simulink model "twotanks_FMINUNC"  (R2017a)
settings: Solver=FixedStepAuto  StartTime=0.0  StopTime=150  FixedStep=0.1  RelTol=1e-3
values from neighbouring files (symbols this model uses):
  q = [1,1]    [MPC_RODAR_PRIMEIRO.m]
  r = [0.0001/(u1^2),0.0001/(u2^2)]    [MPC_RODAR_PRIMEIRO.m]
  Vd = 0.00001*eye(nx)    [MPC_RODAR_PRIMEIRO.m]
  Vn = 0.00001*eye(ny)    [MPC_RODAR_PRIMEIRO.m]
undefined symbols (not defined in the file or in its folder): sysi1, sysi2
libraries: simulink x2
settings Model: Creator=shpac  LastModifiedBy=aguia

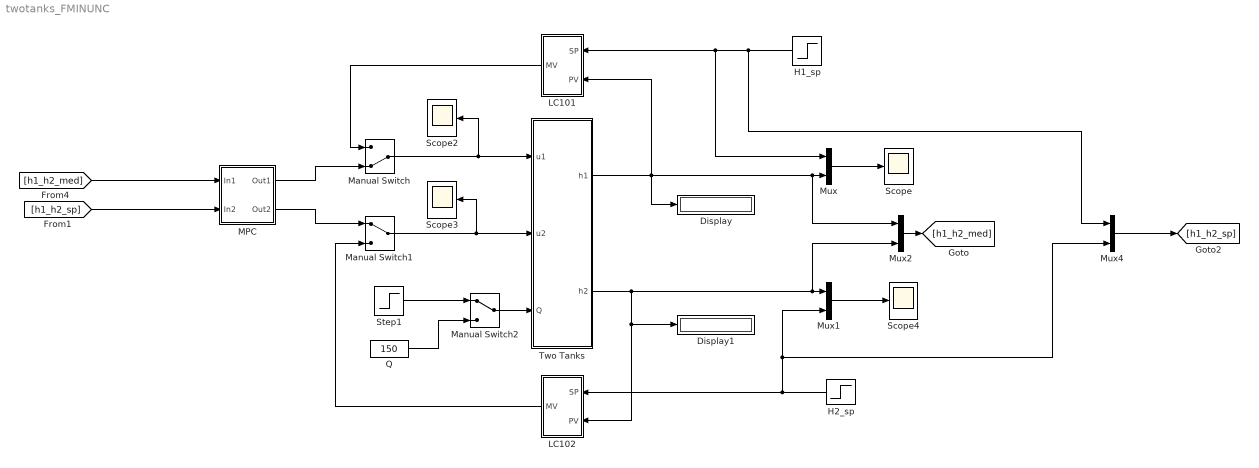
== system twotanks_FMINUNC ==
  Display : Display
  Display1 : Display
  H1_sp : Step  Time=120  Before=0.65  After=0.35  SampleTime=0
  H2_sp : Step  Time=20  Before=0.28  After=0.678  SampleTime=0
  LC101 : Subsystem
  LC102 : Subsystem
  MPC : Subsystem
  Manual Switch : ManualSwitch  CurrentSetting=0
  Manual Switch1 : ManualSwitch
  Manual Switch2 : ManualSwitch
  Mux{,1..2,4} (4 alike) : Mux  Inputs=2
  Q : Constant  Value=150
  Scope{,2..4} (4 alike) : Scope
  Step1 : Step  Time=70  Before=150  After=30  SampleTime=0
  Two Tanks : Subsystem
  wires:
  MPC/1(Out1) -> Manual Switch/2
  [h1_h2_sp] -> MPC/2(In2)
  LC102/1(MV) -> Manual Switch1/2
  Mux/1 -> Scope/1
  Manual Switch2/1 -> Two Tanks/3(Q)
  Mux1/1 -> Scope4/1
  Mux2/1 -> [h1_h2_med]
  LC101/1(MV) -> Manual Switch/1
  Step1/1 -> Manual Switch2/1
  Q/1 -> Manual Switch2/2
  H2_sp/1 -> Mux4/2, Mux1/2, LC102/1(SP)
  Manual Switch/1 -> Scope2/1, Two Tanks/1(u1)
  Two Tanks/2(h2) -> LC102/2(PV), Display1/1, Mux2/2, Mux1/1
  Two Tanks/1(h1) -> Mux2/1, Mux/2, LC101/2(PV), Display/1
  Mux4/1 -> [h1_h2_sp]
  [h1_h2_med] -> MPC/1(In1)
  Manual Switch1/1 -> Scope3/1, Two Tanks/2(u2)
  H1_sp/1 -> Mux4/1, Mux/1, LC101/1(SP)
  MPC/2(Out2) -> Manual Switch1/1

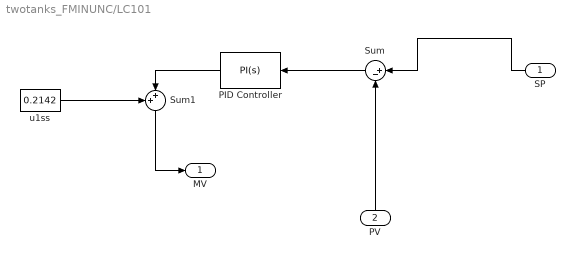
== system twotanks_FMINUNC/LC101 ==
  SP : Inport
  PV : Inport  Port=2
  PID Controller : simulink/Continuous/PID Controller  Controller=PI  TimeDomain=Continuous-time  SampleTime=-1  IntegratorMethod=Forward Euler  FilterMethod=Forward Euler  Form=Ideal  UseFilter=on  ControllerParametersSource=internal  P=-0.667562978885468  I=0.0981942038508327  D=0  N=100  InitialConditionSource=internal  InitialConditionForIntegrator=0  InitialConditionForFilter=0  ExternalReset=none  LimitOutput=on  UpperSaturationLimit=0.7358  LowerSaturationLimit=-0.2042  LinearizeAsGain=on  AntiWindupMode=back-calculation  Kb=1  TrackingMode=off  Kt=1  PParamMin=[]  PParamMax=[]  IParamMin=[]  IParamMax=[]  DParamMin=[]  DParamMax=[]  NParamMin=[]  NParamMax=[]  KbParamMin=[]  KbParamMax=[]  KtParamMin=[]  KtParamMax=[]  POutMin=[]  POutMax=[]  IOutMin=[]  IOutMax=[]  DOutMin=[]  DOutMax=[]  NOutMin=[]  NOutMax=[]  KbOutMin=[]  KbOutMax=[]  KtOutMin=[]  KtOutMax=[]  IntegratorOutMin=[]  IntegratorOutMax=[]  FilterOutMin=[]  FilterOutMax=[]  SumOutMin=[]  SumOutMax=[]  SumI1OutMin=[]  SumI1OutMax=[]  SumI2OutMin=[]  SumI2OutMax=[]  SumI3OutMin=[]  SumI3OutMax=[]  SumDOutMin=[]  SumDOutMax=[]  SaturationOutMin=[]  SaturationOutMax=[]  IntegratorContinuousStateAttributes=''  IntegratorStateMustResolveToSignalObject=off  IntegratorRTWStateStorageClass=Auto  FilterContinuousStateAttributes=''  FilterStateMustResolveToSignalObject=off  FilterRTWStateStorageClass=Auto  DifferentiatorICPrevScaledInput=0  DifferentiatorOutMin=[]  DifferentiatorOutMax=[]  InitialConditionSetting=State (most efficient)
  Sum : Sum  Inputs=|+-
  Sum1 : Sum  Inputs=++|
  u1ss : Constant  Value=0.2142
  MV : Outport
  wires:
  Sum1/1 -> MV/1
  PV/1 -> Sum/2
  PID Controller/1 -> Sum1/2
  SP/1 -> Sum/1
  u1ss/1 -> Sum1/1
  Sum/1 -> PID Controller/1

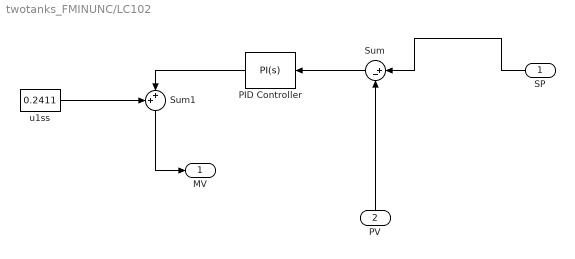
== system twotanks_FMINUNC/LC102 ==
  SP : Inport
  PV : Inport  Port=2
  PID Controller : simulink/Continuous/PID Controller  Controller=PI  TimeDomain=Continuous-time  SampleTime=-1  IntegratorMethod=Forward Euler  FilterMethod=Forward Euler  Form=Ideal  UseFilter=on  ControllerParametersSource=internal  P=-0.11544378631374  I=6.6123973931149  D=0  N=100  InitialConditionSource=internal  InitialConditionForIntegrator=0  InitialConditionForFilter=0  ExternalReset=none  LimitOutput=on  UpperSaturationLimit=0.95-0.2411  LowerSaturationLimit=0.01-0.2411  LinearizeAsGain=on  AntiWindupMode=back-calculation  Kb=1  TrackingMode=off  Kt=1  PParamMin=[]  PParamMax=[]  IParamMin=[]  IParamMax=[]  DParamMin=[]  DParamMax=[]  NParamMin=[]  NParamMax=[]  KbParamMin=[]  KbParamMax=[]  KtParamMin=[]  KtParamMax=[]  POutMin=[]  POutMax=[]  IOutMin=[]  IOutMax=[]  DOutMin=[]  DOutMax=[]  NOutMin=[]  NOutMax=[]  KbOutMin=[]  KbOutMax=[]  KtOutMin=[]  KtOutMax=[]  IntegratorOutMin=[]  IntegratorOutMax=[]  FilterOutMin=[]  FilterOutMax=[]  SumOutMin=[]  SumOutMax=[]  SumI1OutMin=[]  SumI1OutMax=[]  SumI2OutMin=[]  SumI2OutMax=[]  SumI3OutMin=[]  SumI3OutMax=[]  SumDOutMin=[]  SumDOutMax=[]  SaturationOutMin=[]  SaturationOutMax=[]  IntegratorContinuousStateAttributes=''  IntegratorStateMustResolveToSignalObject=off  IntegratorRTWStateStorageClass=Auto  FilterContinuousStateAttributes=''  FilterStateMustResolveToSignalObject=off  FilterRTWStateStorageClass=Auto  DifferentiatorICPrevScaledInput=0  DifferentiatorOutMin=[]  DifferentiatorOutMax=[]  InitialConditionSetting=State (most efficient)
  Sum : Sum  Inputs=|+-
  Sum1 : Sum  Inputs=++|
  u1ss : Constant  Value=0.2411
  MV : Outport
  wires:
  Sum/1 -> PID Controller/1
  u1ss/1 -> Sum1/1
  SP/1 -> Sum/1
  PID Controller/1 -> Sum1/2
  PV/1 -> Sum/2
  Sum1/1 -> MV/1

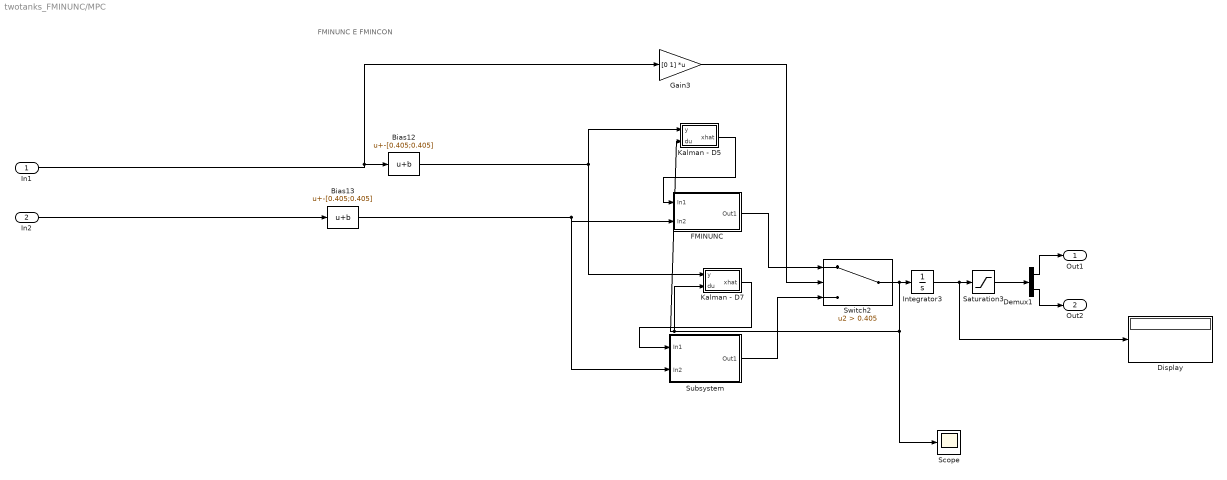
== system twotanks_FMINUNC/MPC ==
  note: FMINUNC E FMINCON
  In1 : Inport
  In2 : Inport  Port=2
  Bias12 : Bias  Bias=-[0.405;0.405]
  Bias13 : Bias  Bias=-[0.405;0.405]
  Demux1 : Demux  Outputs=2
  Display : Display
  FMINUNC : Subsystem
  Gain3 : Gain  Gain=[0 1]  Multiplication=Matrix(K*u)
  Integrator3 : Integrator  InitialCondition=[0.2142;0.2411]
  Kalman - D5 : Subsystem
  Kalman - D7 : Subsystem
  Saturation3 : Saturate  UpperLimit=0.95  LowerLimit=0.01
  Scope : Scope
  Subsystem : Subsystem
  Switch2 : Switch  Criteria=u2 > Threshold  Threshold=0.405
  Out1 : Outport
  Out2 : Outport  Port=2
  wires:
  Kalman - D5/1(xhat) -> FMINUNC/1(In1)
  Kalman - D7/1(xhat) -> Subsystem/1(In1)
  Bias13/1 -> FMINUNC/2(In2), Subsystem/2(In2)
  Bias12/1 -> Kalman - D5/1(y), Kalman - D7/1(y)
  FMINUNC/1(Out1) -> Switch2/1
  Subsystem/1(Out1) -> Switch2/3
  Gain3/1 -> Switch2/2
  Switch2/1 -> Kalman - D7/2(du), Kalman - D5/2(du), Scope/1, Integrator3/1
  Demux1/1 -> Out1/1
  Demux1/2 -> Out2/1
  In1/1 -> Gain3/1, Bias12/1
  In2/1 -> Bias13/1
  Integrator3/1 -> Saturation3/1, Display/1
  Saturation3/1 -> Demux1/1

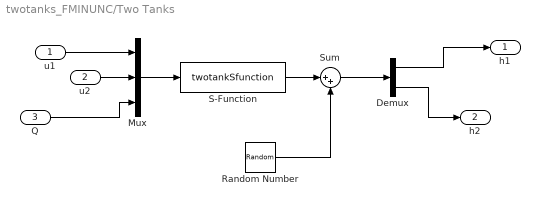
== system twotanks_FMINUNC/Two Tanks ==
  u1 : Inport
  u2 : Inport  Port=2
  Q : Inport  Port=3
  Demux : Demux  Outputs=2
  Mux : Mux  Inputs=3
  Random Number : RandomNumber  Variance=1e-5  SampleTime=0.1
  S-Function : S-Function  FunctionName=twotankSfunction  SFunctionDeploymentMode=off  EnableBusSupport=off
  Sum : Sum  Inputs=|++
  h1 : Outport
  h2 : Outport  Port=2
  wires:
  u2/1 -> Mux/2
  Q/1 -> Mux/3
  Demux/2 -> h2/1
  u1/1 -> Mux/1
  Demux/1 -> h1/1
  Mux/1 -> S-Function/1
  S-Function/1 -> Sum/1
  Sum/1 -> Demux/1
  Random Number/1 -> Sum/2

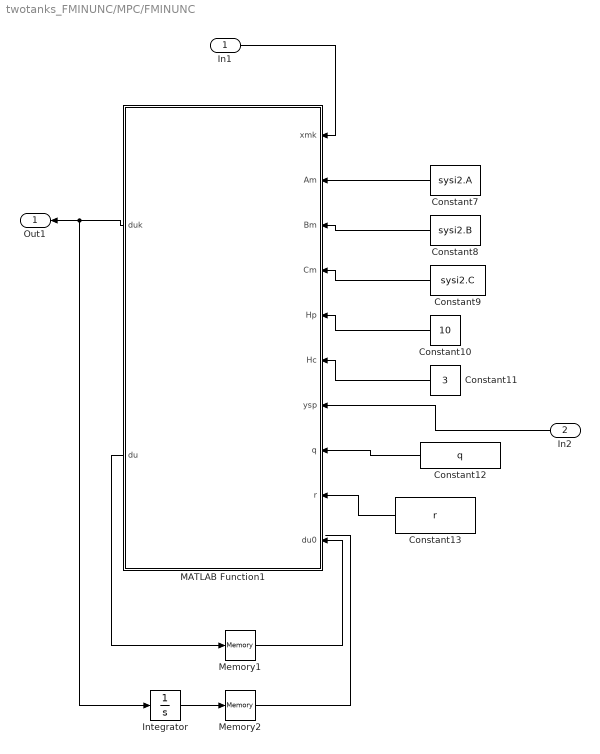
== system twotanks_FMINUNC/MPC/FMINUNC ==
  In1 : Inport
  In2 : Inport  Port=2
  Constant10 : Constant  Value=10
  Constant11 : Constant  Value=3
  Constant12 : Constant  Value=q  VectorParams1D=off
  Constant13 : Constant  Value=r  VectorParams1D=off
  Constant7 : Constant  Value=sysi2.A  VectorParams1D=off
  Constant8 : Constant  Value=sysi2.B  VectorParams1D=off
  Constant9 : Constant  Value=sysi2.C  VectorParams1D=off
  Integrator : Integrator
  MATLAB Function1 : MATLAB Function  TreatAsAtomicUnit=on
  Memory1 : Memory
  Memory2 : Memory
  Out1 : Outport
  wires:
  Memory1/1 -> MATLAB Function1/10(du0)
  Constant11/1 -> MATLAB Function1/6(Hc)
  Constant12/1 -> MATLAB Function1/8(q)
  Constant13/1 -> MATLAB Function1/9(r)
  In1/1 -> MATLAB Function1/1(xmk)
  Constant7/1 -> MATLAB Function1/2(Am)
  MATLAB Function1/2(du) -> Memory1/1
  In2/1 -> MATLAB Function1/7(ysp)
  Constant8/1 -> MATLAB Function1/3(Bm)
  Constant10/1 -> MATLAB Function1/5(Hp)
  MATLAB Function1/1(duk) -> Integrator/1, Out1/1
  Constant9/1 -> MATLAB Function1/4(Cm)
  Memory2/1 -> ?
  Integrator/1 -> Memory2/1

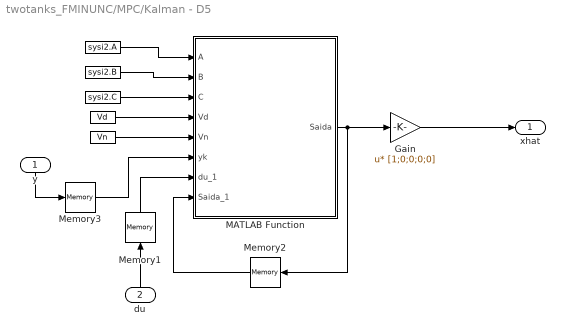
== system twotanks_FMINUNC/MPC/Kalman - D5 ==
  y : Inport
  du : Inport  Port=2
  " " : Constant  Value=sysi2.A
  " " : Constant  Value=sysi2.B
  " " : Constant  Value=sysi2.C
  " " : Constant  Value=Vd
  " " : Constant  Value=Vn
  Gain : Gain  Gain=[1;0;0;0;0]  Multiplication=Matrix(u*K)
  MATLAB Function : MATLAB Function  TreatAsAtomicUnit=on
  Memory1 : Memory  X0=[0;0]
  Memory2 : Memory  X0=[zeros(4,1),Vd]
  Memory3 : Memory  X0=[0;0]
  xhat : Outport
  wires:
  " "/1 -> MATLAB Function/4(Vd)
  " "/1 -> MATLAB Function/1(A)
  " "/1 -> MATLAB Function/5(Vn)
  " "/1 -> MATLAB Function/3(C)
  " "/1 -> MATLAB Function/2(B)
  Memory1/1 -> MATLAB Function/7(du_1)
  Memory3/1 -> MATLAB Function/6(yk)
  Memory2/1 -> MATLAB Function/8(Saida_1)
  Gain/1 -> xhat/1
  MATLAB Function/1(Saida) -> Memory2/1, Gain/1
  du/1 -> Memory1/1
  y/1 -> Memory3/1

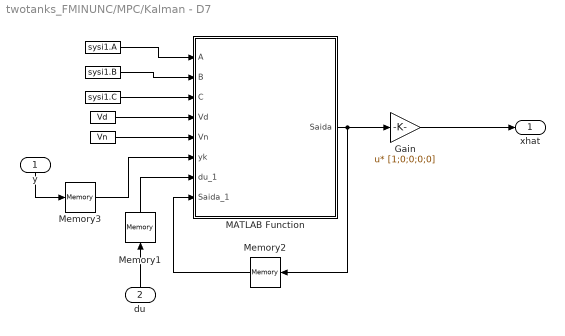
== system twotanks_FMINUNC/MPC/Kalman - D7 ==
  y : Inport
  du : Inport  Port=2
  " " : Constant  Value=sysi1.A
  " " : Constant  Value=sysi1.B
  " " : Constant  Value=sysi1.C
  " " : Constant  Value=Vd
  " " : Constant  Value=Vn
  Gain : Gain  Gain=[1;0;0;0;0]  Multiplication=Matrix(u*K)
  MATLAB Function : MATLAB Function  TreatAsAtomicUnit=on
  Memory1 : Memory  X0=[0;0]
  Memory2 : Memory  X0=[zeros(4,1),Vd]
  Memory3 : Memory  X0=[0;0]
  xhat : Outport
  wires:
  y/1 -> Memory3/1
  du/1 -> Memory1/1
  MATLAB Function/1(Saida) -> Gain/1, Memory2/1
  Gain/1 -> xhat/1
  Memory2/1 -> MATLAB Function/8(Saida_1)
  Memory3/1 -> MATLAB Function/6(yk)
  Memory1/1 -> MATLAB Function/7(du_1)
  " "/1 -> MATLAB Function/2(B)
  " "/1 -> MATLAB Function/3(C)
  " "/1 -> MATLAB Function/5(Vn)
  " "/1 -> MATLAB Function/1(A)
  " "/1 -> MATLAB Function/4(Vd)

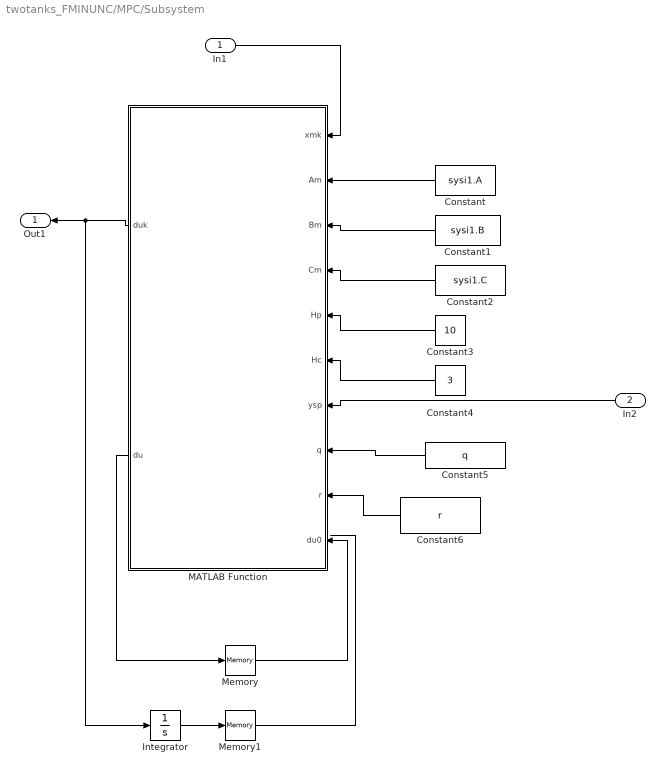
== system twotanks_FMINUNC/MPC/Subsystem ==
  In1 : Inport
  In2 : Inport  Port=2
  Constant : Constant  Value=sysi1.A  VectorParams1D=off
  Constant1 : Constant  Value=sysi1.B  VectorParams1D=off
  Constant2 : Constant  Value=sysi1.C  VectorParams1D=off
  Constant3 : Constant  Value=10
  Constant4 : Constant  Value=3
  Constant5 : Constant  Value=q  VectorParams1D=off
  Constant6 : Constant  Value=r  VectorParams1D=off
  Integrator : Integrator
  MATLAB Function : MATLAB Function  TreatAsAtomicUnit=on
  Memory : Memory
  Memory1 : Memory
  Out1 : Outport
  wires:
  In2/1 -> MATLAB Function/7(ysp)
  Memory/1 -> MATLAB Function/10(du0)
  Constant/1 -> MATLAB Function/2(Am)
  In1/1 -> MATLAB Function/1(xmk)
  Constant4/1 -> MATLAB Function/6(Hc)
  Constant6/1 -> MATLAB Function/9(r)
  Constant1/1 -> MATLAB Function/3(Bm)
  Constant2/1 -> MATLAB Function/4(Cm)
  MATLAB Function/2(du) -> Memory/1
  Constant3/1 -> MATLAB Function/5(Hp)
  Constant5/1 -> MATLAB Function/8(q)
  MATLAB Function/1(duk) -> Integrator/1, Out1/1
  Memory1/1 -> ?
  Integrator/1 -> Memory1/1

== matlab function twotanks_FMINUNC/MPC/Kalman - D5/MATLAB Function ==
  data: A input; B input; C input; Vd input; Vn input; yk input; du_1 input; Saida_1 input; Saida output
function Saida = fcn(A, B, C, Vd, Vn, yk, du_1, Saida_1 )
    nx = length(A);
    xmk = Saida_1(:,1);
    P = Saida_1(:,2:end);
    % Filtro de kalman - predicao
    xmk = (A)*xmk + B*(du_1);
    ymk = C*xmk;
    P = A*P*A' + Vd;
    % Filtro de Kalman - correcao
    K = P*C'/(C*P*C' + Vn);
    xmk = xmk + K*(yk - ymk);
    P = (eye(nx) - K*C)*P;
    Saida = [xmk,P];

== matlab function twotanks_FMINUNC/MPC/Kalman - D7/MATLAB Function ==
  data: A input; B input; C input; Vd input; Vn input; yk input; du_1 input; Saida_1 input; Saida output
function Saida = fcn(A, B, C, Vd, Vn, yk, du_1, Saida_1 )
    nx = length(A);
    xmk = Saida_1(:,1);
    P = Saida_1(:,2:end);
    % Filtro de kalman - predicao
    xmk = (A)*xmk + B*(du_1);
    ymk = C*xmk;
    P = A*P*A' + Vd;
    % Filtro de Kalman - correcao
    K = P*C'/(C*P*C' + Vn);
    xmk = xmk + K*(yk - ymk);
    P = (eye(nx) - K*C)*P;
    Saida = [xmk,P];

== matlab function twotanks_FMINUNC/MPC/Subsystem/MATLAB Function ==
  data: xmk input; Am input; Bm input; Cm input; Hp input; Hc input; ysp input; q input; r input; duk output; du0 input; du output
function [duk, du] = MPC_twotanks_simulink(xmk, Am, Bm, Cm, Hp, Hc, ysp, q, r, du0)

coder.extrinsic('MPC_twotanks')

sysi.A = Am;
sysi.B = Bm;
sysi.C = Cm;

nu = size(sysi.B,2) ;

duk = [0 ; 0];

du = ones(6,1) ;
    
[du, duk] = MPC_twotanks(xmk, Am, Bm, Cm, Hp, Hc, ysp, q, r, du0) ;

end

== matlab function twotanks_FMINUNC/MPC/FMINUNC/MATLAB Function1 ==
  data: xmk input; Am input; Bm input; Cm input; Hp input; Hc input; ysp input; q input; r input; duk output; du0 input; du output
function [duk, du] = MPC_twotanks_simulink(xmk, Am, Bm, Cm, Hp, Hc, ysp, q, r, du0)

coder.extrinsic('MPC_twotanks')

sysi.A = Am;
sysi.B = Bm;
sysi.C = Cm;

nu = size(sysi.B,2) ;

duk = [0 ; 0];

du = ones(6,1) ;
    
[du, duk] = MPC_twotanks(xmk, Am, Bm, Cm, Hp, Hc, ysp, q, r, du0) ;

end
